simulink model "Compare_Test"  (R2014b)
settings: Solver=ode45  StartTime=0.0  StopTime=inf  MaxStep=0.001  RelTol=1e-3
libraries: simulink x2
settings Model: Creator=INTEL  LastModifiedBy=INTEL

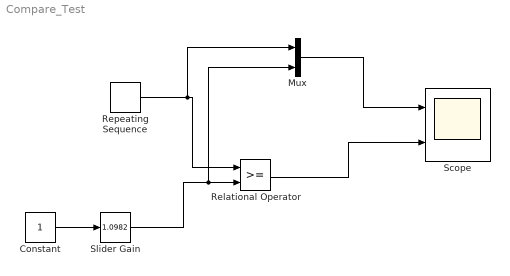
== system Compare_Test ==
  Constant : Constant
  Mux : Mux  Inputs=2
  Relational Operator : RelationalOperator  OutDataTypeStr=boolean
  Repeating Sequence : simulink/Sources/Repeating Sequence  rep_seq_t=[0 0.01 0.02]  rep_seq_y=[0 2 0]
  Scope : Scope  NumInputPorts=2
      settings: TimeRange=0.04  YMin=-1~-1  YMax=3~2
  Slider Gain : simulink/Math Operations/Slider Gain  low=0  gain=1.0982  high=2
  wires:
  Repeating Sequence/1 -> Mux/1, Relational Operator/1
  Mux/1 -> Scope/1
  Relational Operator/1 -> Scope/2
  Constant/1 -> Slider Gain/1
  Slider Gain/1 -> Mux/2, Relational Operator/2
